simulink model "PlantaSavePointPneuLongitudinalComCalculoVT"  (R2024b)
settings: Solver=ode23tb  StartTime=0.0  StopTime=100  MaxStep=0.01  RelTol=2e-3
values from neighbouring files (symbols this model uses):
  C1 = 1.2801    [CodigoSavePoint.m]    (also in CodigoVT.m)
  C2 = 23.99    [CodigoSavePoint.m]    (also in CodigoVT.m)
  C3 = 0.52    [CodigoSavePoint.m]    (also in CodigoVT.m)
undefined symbols (not defined in the file or in its folder): EV, MTR
libraries: autolibshared x5, slpidlib x2, autolibmappedmotor x2, vrlib x1, vehdynlibviscommon x1, vehdynlibscenariocommon x1, vehdynlibsteering x1, vehdynlibdriver x1
(part 1 of 4)
settings Model: Creator=João Gabriel  LastModifiedBy=João Gabriel
settings SolverCC: ZeroCrossAlgorithm=Adaptive  AutoInsertRateTranBlk=on  InsertRTBMode=Never (minimum delay)
settings DebuggingCC: IgnoredZcDiagnostic=none  UnderSpecifiedDimensionMsg=warning
settings ModelReferenceCC: EnableParallelModelReferenceBuilds=on  ModelReferenceMinAlgLoopOccurrences=on  PropagateSignalLabelsOutOfModel=off

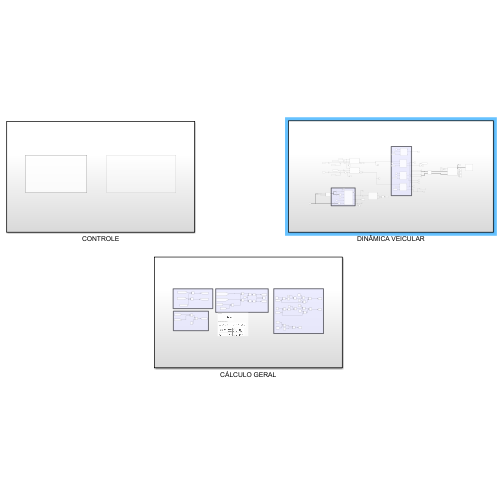
[thumbnail: Simulink's stored preview of the top-level diagram]
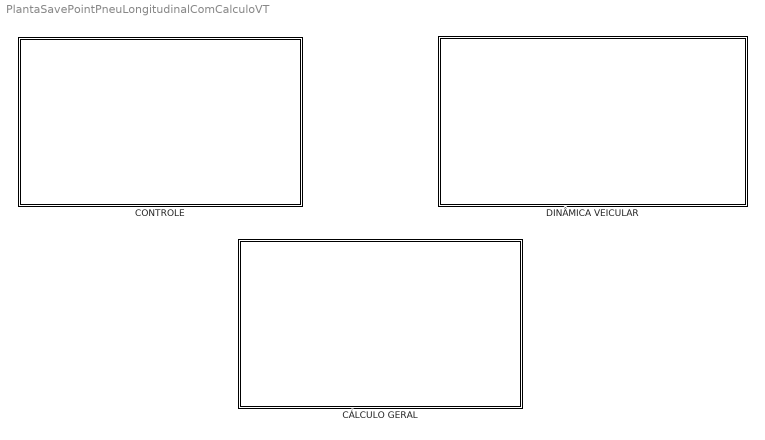
== system PlantaSavePointPneuLongitudinalComCalculoVT ==
  CONTROLE : Subsystem
  CÁLCULO GERAL : Subsystem
  DINÂMICA VEICULAR : Subsystem

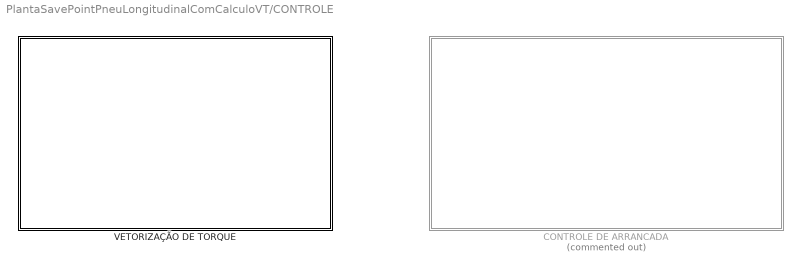
== system PlantaSavePointPneuLongitudinalComCalculoVT/CONTROLE ==
  "CONTROLE DE ARRANCADA " : Subsystem  Commented=on
  "VETORIZAÇÃO DE TORQUE " : Subsystem

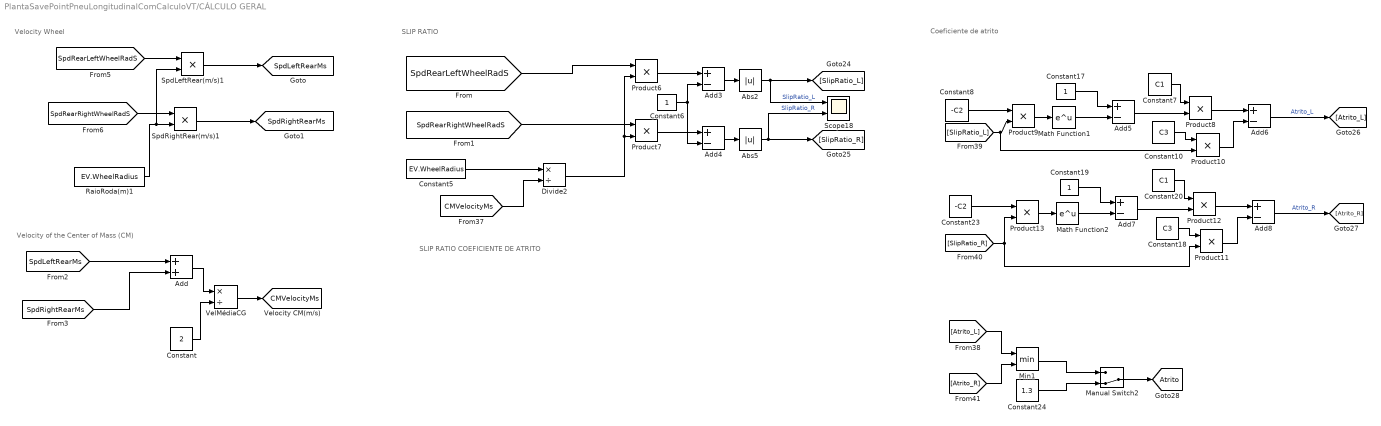
== system PlantaSavePointPneuLongitudinalComCalculoVT/CÁLCULO GERAL ==
  note: Coeficiente de atrito
  note: SLIP RATIO
      |
      | COEFICIENTE DE ATRITO
  note: SLIP RATIO
  note: Velocity Wheel
  note: Velocity of the Center of Mass (CM)
  Abs2 : Abs  SaturateOnIntegerOverflow=off
  Abs5 : Abs  SaturateOnIntegerOverflow=off
  Add : Sum
  Add{3..8} (6 alike) : Sum  Inputs=+-
  Constant : Constant  Value=2
  Constant10 : Constant  Value=C3
  Constant17 : Constant
  Constant18 : Constant  Value=C3
  Constant19 : Constant
  Constant20 : Constant  Value=C1
  Constant23 : Constant  Value=-C2
  Constant24 : Constant  Value=1.3
  Constant5 : Constant  Value=EV.WheelRadius  VectorParams1D=off
  Constant6 : Constant
  Constant7 : Constant  Value=C1
  Constant8 : Constant  Value=-C2
  Divide2 : Product  Inputs=*/
  Manual Switch2 : ManualSwitch  CurrentSetting=0
  Math Function1 : Math
  Math Function2 : Math
  Min1 : MinMax  Inputs=2
  Product{6..13} (8 alike) : Product
  RaioRoda(m)1 : Constant  Value=EV.WheelRadius  VectorParams1D=off
  Scope18 : Scope  NumInputPorts=2
  SpdLeftRear(m/s)1 : Product
  SpdRightRear(m/s)1 : Product
  VelMédiaCG : Product  Inputs=*/
  tag scope: Atrito=global, CMVelocityMs=global, SpdLeftRearMs=global, SpdRightRearMs=global
  wires:
  Add6/1 -> [Atrito_L]  "Atrito_L"
  Constant7/1 -> Product8/1
  Constant19/1 -> Add7/1
  Constant24/1 -> Manual Switch2/2
  Constant23/1 -> Product13/1
  Product11/1 -> Add8/2
  Product12/1 -> Add8/1
  Product10/1 -> Add6/2
  Product8/1 -> Add6/1
  Math Function2/1 -> Add7/2
  Add7/1 -> Product12/2
  [Atrito_L] -> Min1/1
  Constant10/1 -> Product10/1
  Math Function1/1 -> Add5/2
  Constant18/1 -> Product11/1
  [SlipRatio_L] -> Product10/2, Product9/2
  Add8/1 -> [Atrito_R]  "Atrito_R"
  Product9/1 -> Math Function1/1
  Min1/1 -> Manual Switch2/1
  Constant8/1 -> Product9/1
  Constant17/1 -> Add5/1
  [Atrito_R] -> Min1/2
  Product13/1 -> Math Function2/1
  Constant20/1 -> Product12/1
  Add5/1 -> Product8/2
  [SlipRatio_R] -> Product13/2, Product11/2
  Manual Switch2/1 -> [Atrito]
  Constant6/1 -> Add3/2, Add4/2
  [SpdRearRightWheelRadS] -> Product7/1
  Abs5/1 -> Scope18/2, [SlipRatio_R]  "SlipRatio_R"
  [CMVelocityMs] -> Divide2/2
  Divide2/1 -> Product6/2, Product7/2
  Add3/1 -> Abs2/1
  Add4/1 -> Abs5/1
  Product7/1 -> Add4/1
  [SpdRearLeftWheelRadS] -> Product6/1
  Product6/1 -> Add3/1
  Constant5/1 -> Divide2/1
  Abs2/1 -> Scope18/1, [SlipRatio_L]  "SlipRatio_L"
  [SpdRearLeftWheelRadS] -> SpdLeftRear(m/s)1/1
  SpdRightRear(m/s)1/1 -> [SpdRightRearMs]
  SpdLeftRear(m/s)1/1 -> [SpdLeftRearMs]
  RaioRoda(m)1/1 -> SpdLeftRear(m/s)1/2, SpdRightRear(m/s)1/2
  [SpdRearRightWheelRadS] -> SpdRightRear(m/s)1/1
  Constant/1 -> VelMédiaCG/2
  [SpdLeftRearMs] -> Add/1
  [SpdRightRearMs] -> Add/2
  Add/1 -> VelMédiaCG/1
  VelMédiaCG/1 -> [CMVelocityMs]
